simulink model "child"  (R2023b)
settings: Solver=FixedStepDiscrete  StartTime=0.0  StopTime=10.0  FixedStep=1e-2  RelTol=1e-3
libraries: simulink x2
settings Model: Creator=mfussi  LastModifiedBy=mfussi
settings OptimizationCC: DefaultParameterBehavior=Inlined  EnhancedBackFolding=on  PassReuseOutputArgsAs=Individual arguments  ZeroExternalMemoryAtStartup=off  ZeroInternalMemoryAtStartup=off  OptimizeBlockOrder=speed  DifferentSizesBufferReuse=on  OptimizationCustomize=off  EfficientTunableParamExpr=on
settings DebuggingCC: ParameterTunabilityLossMsg=error
settings SFSimCC: MATLABDynamicMemAlloc=off
settings RTWCC: Description=Embedded Coder  SystemTargetFile=ert.tlc  TemplateMakefile=ert_default_tmf
settings CodeAppCC: ForceParamTrailComments=on  IgnoreCustomStorageClasses=off  OperatorAnnotations=on  SimulinkDataObjDesc=on  SFDataObjDesc=on  InsertBlockDesc=on
settings ERTTargetCC: TargetLangStandard=C99 (ISO)  GenerateSampleERTMain=on  InlinedParameterPlacement=NonHierarchical  ERTCustomFileTemplate=example_file_process.tlc

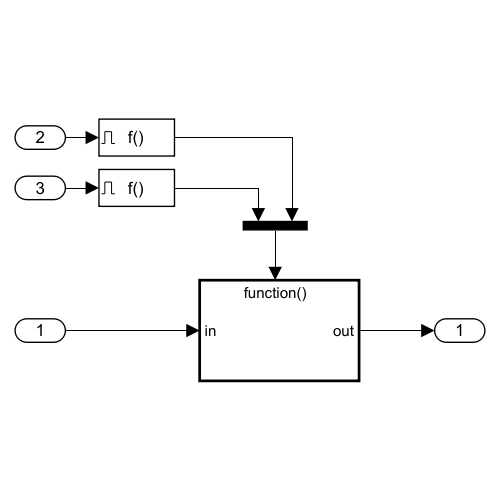
[thumbnail: Simulink's stored preview of the top-level diagram]
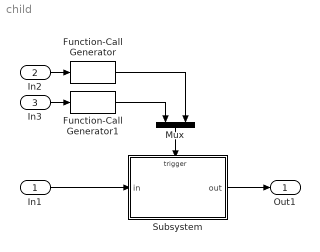
== system child ==
  In1 : Inport
  In2 : Inport  Port=2
  In3 : Inport  Port=3
  Function-Call Generator : simulink/Ports & Subsystems/Function-Call Generator  sample_time=1  numberOfIterations=1  DisallowWideOutput=off  ShowEnablePort=on
  Function-Call Generator1 : simulink/Ports & Subsystems/Function-Call Generator  sample_time=1  numberOfIterations=1  DisallowWideOutput=off  ShowEnablePort=on
  Mux : Mux  Inputs=2
  Subsystem : Subsystem
  Out1 : Outport
  wires:
  In1/1 -> Subsystem/1(in)
  Subsystem/1(out) -> Out1/1
  In2/1 -> Function-Call Generator/1
  Function-Call Generator/1 -> Mux/2
  In3/1 -> Function-Call Generator1/1
  Function-Call Generator1/1 -> Mux/1
  Mux/1 -> Subsystem/Trigger

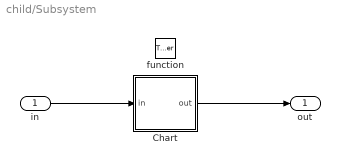
== system child/Subsystem ==
  in : Inport
  function : TriggerPort  TriggerType=function-call  VariantControl=(inherit)
  Chart : Stateflow chart  TreatAsAtomicUnit=on
  out : Outport
  wires:
  in/1 -> Chart/1(in)
  Chart/1(out) -> out/1

== stateflow chart child/Subsystem/Chart ==
  state Tick
    entry:
    out = 0.5 * in;
  state Tock
    entry:
    out = 1 * in;
  (default) -> Tick
  Tick -> Tock : after(0.1,sec)
  Tock -> Tick : after(0.1,sec)
  data: in input; out output
